simulink subsystem "Losses_calculation"  (R2024a)
settings: Solver=VariableStepAuto  StartTime=0.0  StopTime=10.0  RelTol=1e-3
undefined symbols (not defined in the file): DCDC, rd, rl, ron, Vd
settings Model: Creator=Henrique Mesquita  LastModifiedBy=henri

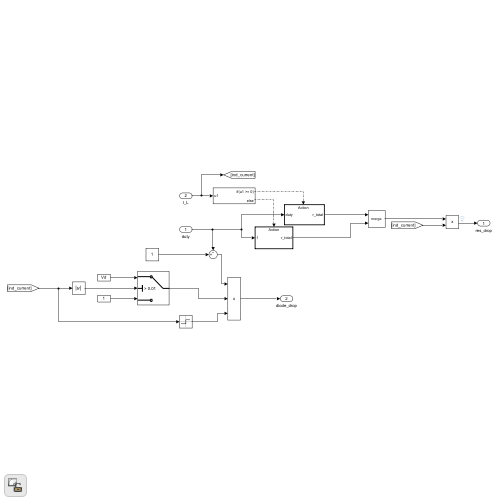
[thumbnail: Simulink's stored preview of the top-level diagram]
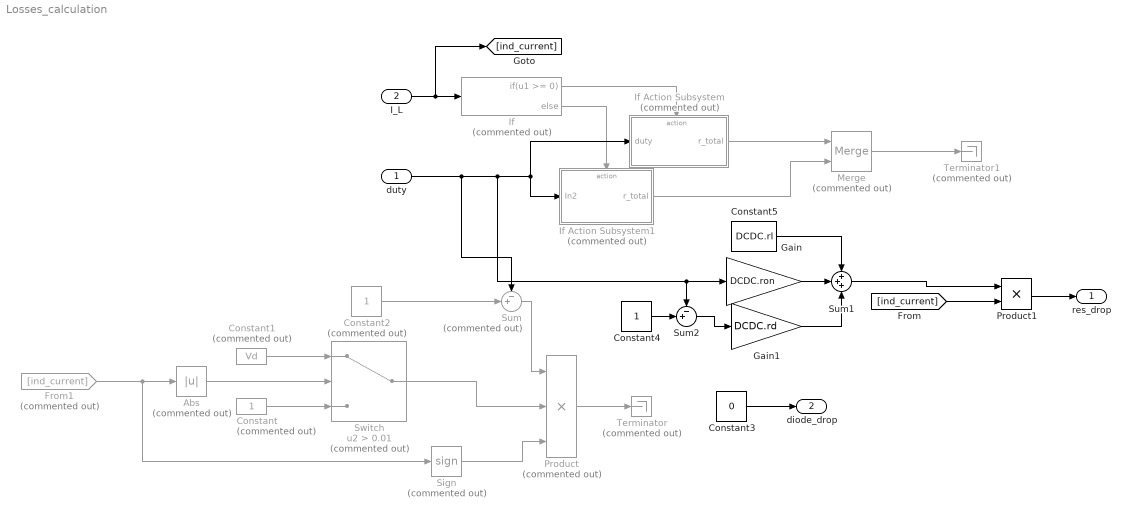
== system Losses_calculation ==
  duty : Inport
  I_L : Inport  Port=2
  Abs : Abs  Commented=on  SaturateOnIntegerOverflow=off
  Constant : Constant  Commented=on
  Constant1 : Constant  Commented=on  Value=Vd
  Constant2 : Constant  Commented=on
  Constant3 : Constant  Value=0
  Constant4 : Constant
  Constant5 : Constant  Value=DCDC.rl
  From1 : From  Commented=on  GotoTag=ind_current
  Gain : Gain  Gain=DCDC.ron
  Gain1 : Gain  Gain=DCDC.rd
  If : If  Commented=on  IfExpression=u1 >= 0
  If Action Subsystem : Subsystem  Commented=on  TreatAsAtomicUnit=on
  If Action Subsystem1 : Subsystem  Commented=on  TreatAsAtomicUnit=on
  Merge : Merge  Commented=on
  Product : Product  Commented=on  Inputs=3
  Product1 : Product
  Sign : Signum  Commented=on
  Sum : Sum  Commented=on  Inputs=-+|
  Sum1 : Sum  Inputs=+++
  Sum2 : Sum  Inputs=-+|
  Switch : Switch  Commented=on  Criteria=u2 > Threshold  Threshold=0.01  SaturateOnIntegerOverflow=off  InputSameDT=off
  Terminator : Terminator  Commented=on
  Terminator1 : Terminator  Commented=on
  res_drop : Outport
  diode_drop : Outport  Port=2
  wires:
  Switch/1 -> Product/2
  Product/1 -> Terminator/1
  Sign/1 -> Product/3
  Constant/1 -> Switch/3
  From1/1 -> Sign/1, Abs/1
  Sum/1 -> Product/1
  If/2 -> If Action Subsystem1/Action
  [ind_current] -> Product1/2
  If Action Subsystem/1(r_total) -> Merge/1
  Constant2/1 -> Sum/2
  Product1/1 -> res_drop/1
  Abs/1 -> Switch/2
  If/1 -> If Action Subsystem/Action
  Merge/1 -> Terminator1/1
  If Action Subsystem1/1(r_total) -> Merge/2
  I_L/1 -> If/1, [ind_current]
  Constant1/1 -> Switch/1
  Constant3/1 -> diode_drop/1
  Constant4/1 -> Sum2/2
  Gain1/1 -> Sum1/3
  Constant5/1 -> Sum1/1
  Sum2/1 -> Gain1/1
  duty/1 -> If Action Subsystem/1(duty), If Action Subsystem1/1(In2), Gain/1, Sum2/1, Sum/1
  Sum1/1 -> Product1/1
  Gain/1 -> Sum1/2

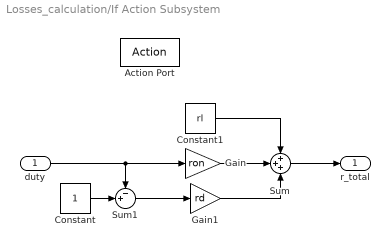
== system Losses_calculation/If Action Subsystem ==
  duty : Inport
  Action Port : ActionPort
  Constant : Constant
  Constant1 : Constant  Value=rl
  Gain : Gain  Gain=ron
  Gain1 : Gain  Gain=rd
  Sum : Sum  Inputs=+++
  Sum1 : Sum  Inputs=-+|
  r_total : Outport
  wires:
  Constant/1 -> Sum1/2
  Sum1/1 -> Gain1/1
  Constant1/1 -> Sum/1
  Gain1/1 -> Sum/3
  duty/1 -> Gain/1, Sum1/1
  Gain/1 -> Sum/2
  Sum/1 -> r_total/1

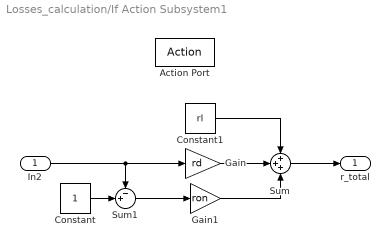
== system Losses_calculation/If Action Subsystem1 ==
  In2 : Inport
  Action Port : ActionPort
  Constant : Constant
  Constant1 : Constant  Value=rl
  Gain : Gain  Gain=rd
  Gain1 : Gain  Gain=ron
  Sum : Sum  Inputs=+++
  Sum1 : Sum  Inputs=-+|
  r_total : Outport
  wires:
  Sum1/1 -> Gain1/1
  Sum/1 -> r_total/1
  Constant/1 -> Sum1/2
  Constant1/1 -> Sum/1
  Gain/1 -> Sum/2
  Gain1/1 -> Sum/3
  In2/1 -> Gain/1, Sum1/1
